simulink model "Counter1"  (R2016a)
settings: Solver=FixedStepDiscrete  StartTime=0.0  StopTime=10.0  RelTol=1e-3
settings Model: Creator=Mohamed Fawzy  LastModifiedBy=Mohamed Fawzy
settings OptimizationCC: DefaultParameterBehavior=Inlined  OptimizeModelRefInitCode=on  LifeSpan=1
settings RTWCC: SystemTargetFile=ert.tlc  GenCodeOnly=on  GenerateMakefile=off  TemplateMakefile=ert_default_tmf  GenerateReport=on  IncludeHyperlinkInReport=on  LaunchReport=on  GenerateTraceInfo=on  GenerateTraceReport=on  GenerateTraceReportSl=on  GenerateTraceReportSf=on  GenerateTraceReportEml=on
settings CodeAppCC: ForceParamTrailComments=on  IgnoreCustomStorageClasses=off  OperatorAnnotations=on  SimulinkDataObjDesc=on  SFDataObjDesc=on  MATLABFcnDesc=on  InsertBlockDesc=on  MATLABSourceComments=on
settings ERTTargetCC: GenerateSampleERTMain=on  SuppressErrorStatus=on  InlinedParameterPlacement=NonHierarchical  ERTCustomFileTemplate=example_file_process.tlc

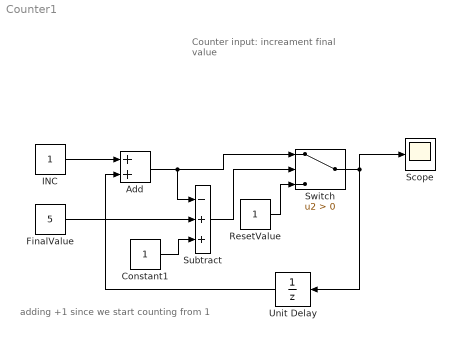
== system Counter1 ==
  note: adding +1 since we start counting from 1
  note: Counter
      |
      | input:
      | increament
      | final value
  Add : Sum  AccumDataTypeStr=uint8
  Constant1 : Constant  OutDataTypeStr=uint8
  FinalValue : Constant  Value=5  OutDataTypeStr=uint8
  INC : Constant  OutDataTypeStr=uint8
  "ResetValue " : Constant  OutDataTypeStr=uint8
  Scope : Scope
  Subtract : Sum  Inputs=-++  AccumDataTypeStr=uint8
  Switch : Switch  Criteria=u2 > Threshold  OutDataTypeStr=uint8
  Unit Delay : UnitDelay  SampleTime=-1
  wires:
  INC/1 -> Add/1
  Switch/1 -> Scope/1, Unit Delay/1
  Unit Delay/1 -> Add/2
  Add/1 -> Subtract/1, Switch/1
  Subtract/1 -> Switch/2
  "ResetValue "/1 -> Switch/3
  FinalValue/1 -> Subtract/2
  Constant1/1 -> Subtract/3
